simulink model "SAS_noSAS"  (R2016b)
settings: Solver=VariableStepAuto  StartTime=0.0  StopTime=10.0  RelTol=1e-3
values from neighbouring files (symbols this model uses):
  actua = ss(aa,ba,ca,da,            'name'      ,'Actuator',            'StateName' ,{ 'xda' , 'xdr' },            'StateUnit' ,{'[rad]','[rad]'},            'InputName' ,{ 'ua'  , 'ur'  },            'InputUnit' ,{'[rad]','[rad]'},            'OutputName',{ 'da'  , 'dr'  },            'OutputUnit',{'[rad]','[rad]'})    [Roll_Yaw_Damper_Design.m]
  kp = 0.4    [Roll_Yaw_Damper_Design.m]
  kr = 1.3    [Roll_Yaw_Damper_Design.m]
  plant = ss(ap,bp,cp,dp,      'name'     ,'Longitudinal Dynamic F16',      'StateName',{'beta' , 'phi' ,   'p'   ,   'r'   },      'StateUnit',{'[rad]','[rad]','[rad/s]','[rad/s]'},      'InputName',{ 'da'  , 'dr'  },      'InputUnit',{'[rad]','[rad]'},      'OutputName',{   'p'   ,  'r'},      'OutputUnit',{'[deg/s]','[deg/s]'})    [Roll_Yaw_Damper_Design.m]
  wash = ss(aw,bw,cw,dw,        'name'      ,'wash-out filter',        'StateName' ,{  'xw'   },        'StateUnit' ,{'[deg/s]'},        'InputName' ,{   'p'   ,   'r'   },        'InputUnit' ,{'[deg/s]','[deg/s]'},        'OutputName',{ 'pw'  , 'rw'  },        'OutputUnit',{'[deg/s]','[deg/s]'})    [Roll_Yaw_Damper_Design.m]
undefined symbols (not defined in the file or in its folder): sigbuilder_block
settings Model: Creator=Gianni  LastModifiedBy=Gianni

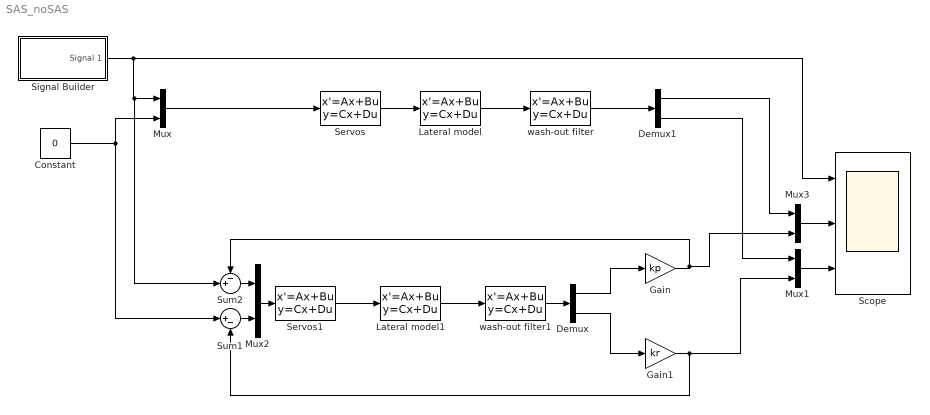
== system SAS_noSAS ==
  Constant : Constant  Value=0
  Demux : Demux  Outputs=2
  Demux1 : Demux  Outputs=2
  Gain : Gain  Gain=kp
  Gain1 : Gain  Gain=kr
  Lateral model : StateSpace  A=plant.a  B=plant.b  C=plant.c  D=plant.d  X0=0
  Lateral model1 : StateSpace  A=plant.a  B=plant.b  C=plant.c  D=plant.d  X0=0
  Mux{,1..3} (4 alike) : Mux  Inputs=2
  Scope : Scope  NumInputPorts=3
  Servos : StateSpace  A=actua.a  B=actua.b  C=actua.c  D=actua.d  X0=0
  Servos1 : StateSpace  A=actua.a  B=actua.b  C=actua.c  D=actua.d  X0=0
  Signal Builder : Subsystem  Tag=STV Subsys  LoadFcn=sigbuilder_block('load');  StartFcn=sigbuilder_block('start');  StopFcn=sigbuilder_block('stop');  ClipboardFcn=sigbuilder_block('clipboard');  mask(Sigbuilder block){tuvar=[0:10]}
      mask help: Simulink:masks:SigbuilderBlock_MD
      mask init:
      | if ~strcmp(get_param(bdroot(gcbh),'SimulationStatus'),'stopped') tuvar = sigbuilder_block('maskInit'); end
      settings: CopyFcn=sigbuilder_block('copy');  DeleteFcn=sigbuilder_block('delete');  ModelCloseFcn=sigbuilder_block('modelClose');  PreSaveFcn=sigbuilder_block('preSave');  PauseFcn=sigbuilder_block('pause');  ContinueFcn=sigbuilder_block('continue');  NameChangeFcn=sigbuilder_block('namechange');  OpenFcn=sigbuilder_block('open',[118.5 207 550.5 399.75 ]);  CloseFcn=sigbuilder_block('close');
      mask Display: plot(0, 0, 100, 100,[2, 2, 32, 32, 2], [68, 8, 8, 68, 68],[32, 2], [38, 38], [32, 19, 2],[53, 60, 44], [32, 17, 17, 2],[16, 16, 31, 31]);txt = getActiveGroup(gcbh);text(2, 100, txt,'verticalAlignment', 'top');
  Sum1 : Sum  Inputs=|+-
  Sum2 : Sum  Inputs=-+|
  wash-out filter : StateSpace  A=wash.a  B=wash.b  C=wash.c  D=wash.d  X0=0
  wash-out filter1 : StateSpace  A=wash.a  B=wash.b  C=wash.c  D=wash.d  X0=0
  wires:
  Lateral model/1 -> wash-out filter/1
  Servos/1 -> Lateral model/1
  Mux/1 -> Servos/1
  Constant/1 -> Sum1/1, Mux/2
  wash-out filter/1 -> Demux1/1
  Servos1/1 -> Lateral model1/1
  Lateral model1/1 -> wash-out filter1/1
  wash-out filter1/1 -> Demux/1
  Demux/1 -> Gain/1
  Demux/2 -> Gain1/1
  Sum2/1 -> Mux2/1
  Mux2/1 -> Servos1/1
  Sum1/1 -> Mux2/2
  Gain/1 -> Mux3/2, Sum2/1
  Signal Builder/1(Signal 1) -> Sum2/2, Mux/1, Scope/1
  Mux1/1 -> Scope/3
  Gain1/1 -> Mux1/2, Sum1/2
  Demux1/2 -> Mux1/1
  Mux3/1 -> Scope/2
  Demux1/1 -> Mux3/1

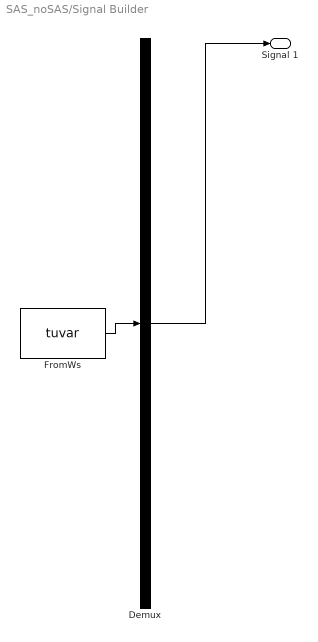
== system SAS_noSAS/Signal Builder ==
  Demux : Demux  Tag=STV Demux  Outputs=1
  FromWs : FromWorkspace  Tag=STV FromWs  VariableName=tuvar  SampleTime=0
      SigBuilderData=|
      | common.afterFinalStr = 'Extrapolate'
      | common.sampleTime = 0
      | dataSet.timeRange = [0 10]
      | dataSet.name = 'Group 1'
      | sbobj.Groups.Name = 'Group 1'
      | sbobj.Groups.Signals.Name = 'Signal 1'
      | sbobj.Groups.Signals.XData = [0 1 1 3 3 5 5 10]
      | sbobj.Groups.Signals.YData = [0 0 1 1 -1 -1 0 0]
  Signal 1 : Outport  Tag=STV Outport
  wires:
  Demux/1 -> Signal 1/1
  FromWs/1 -> Demux/1
